simulink model "simexa26"  (Simulink 2.09)
settings: Solver=ode45  StartTime=0.0  StopTime=10  RelTol=1e-3  AbsTol=1e-6
settings Model: ConsistencyChecking=off  RTWTemplateMakefile=grt_vc.tmf

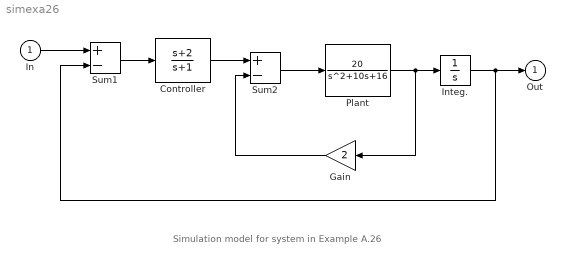
== system simexa26 ==
  note: Simulation model for system in Example A.26
  In : Inport  Port=1  PortWidth=-1  SampleTime=-1
  Controller : TransferFcn  Numerator=[1 2]  Denominator=[1 1]
  Gain : Gain  Orientation=left  Gain=2
  Integ. : Integrator  ExternalReset=none  InitialConditionSource=internal  InitialCondition=0  LimitOutput=off  UpperSaturationLimit=inf  LowerSaturationLimit=-inf  ShowSaturationPort=off  ShowStatePort=off  AbsoluteTolerance=auto
  Plant : TransferFcn  Numerator=[20]  Denominator=[1 10 16]
  Sum1 : Sum  Inputs=+-
  Sum2 : Sum  Inputs=+-
  Out : Outport  Port=1  InitialOutput=0
  wires:
  Integ./1 -> Sum1/2, Out/1
  In/1 -> Sum1/1
  Controller/1 -> Sum2/1
  Sum1/1 -> Controller/1
  Plant/1 -> Gain/1, Integ./1
  Gain/1 -> Sum2/2
  Sum2/1 -> Plant/1
